simulink subsystem "INA219_Voltage_Sensor"  (R2022b)
settings: Solver=VariableStepAuto  StartTime=0.0  StopTime=10.0  RelTol=1e-3
undefined symbols (not defined in the file): INA219
settings Model: Creator=gotta  LastModifiedBy=gotta

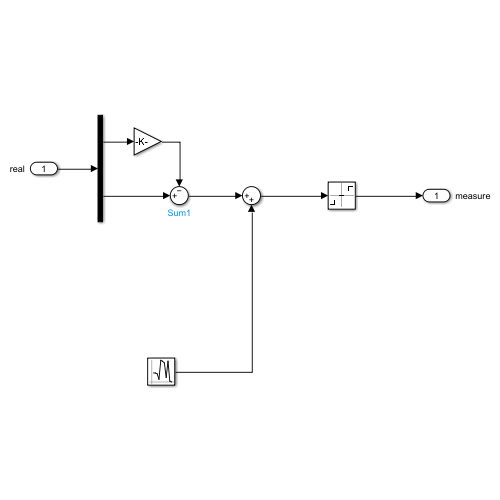
[thumbnail: Simulink's stored preview of the top-level diagram]
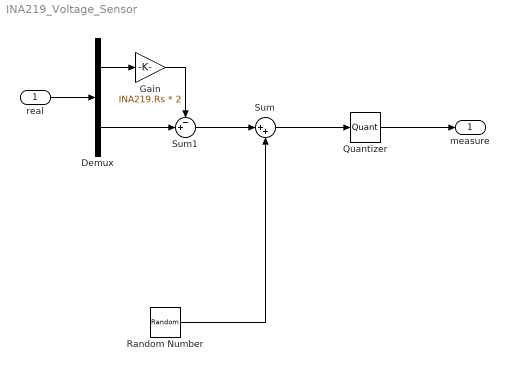
== system INA219_Voltage_Sensor ==
  real : Inport
  Demux : Demux  Outputs=2
  Gain : Gain  Gain=INA219.Rs * 2
  Quantizer : Quantizer  QuantizationInterval=INA219.Vstep
  Random Number : RandomNumber  Variance=2.5e-3  SampleTime=1e-3
  Sum : Sum  Inputs=|++
  Sum1 : Sum  Inputs=-+|
  measure : Outport
  wires:
  Sum/1 -> Quantizer/1
  real/1 -> Demux/1
  Quantizer/1 -> measure/1
  Random Number/1 -> Sum/2
  Demux/2 -> Sum1/2
  Demux/1 -> Gain/1
  Gain/1 -> Sum1/1
  Sum1/1 -> Sum/1
